simulink model "diagb"  (R2015a)
settings: Solver=ode45  StartTime=0.0  StopTime=10.0  RelTol=1e-3
settings Model: Creator=dayanm  LastModifiedBy=HP-14
settings OptimizationCC: ExpressionDepthLimit=2147483647
settings DebuggingCC: UnderspecifiedInitializationDetection=Classic  MergeDetectMultiDrivingBlocksExec=none  SolverPrmCheckMsg=warning  StateNameClashWarn=warning

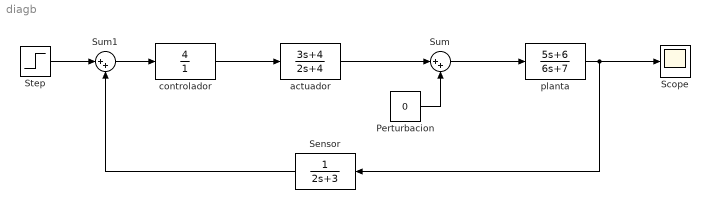
== system diagb ==
  Perturbacion : Constant  Value=0
  Scope : Scope
  Sensor : TransferFcn  Denominator=[2 3]
  Step : Step  SampleTime=0
  Sum : Sum  Inputs=|++
  Sum1 : Sum  Inputs=|++
  actuador : TransferFcn  Numerator=[3 4]  Denominator=[2 4]
  controlador : TransferFcn  Numerator=[4 ]  Denominator=[1]
  planta : TransferFcn  Numerator=[5 6]  Denominator=[6 7]
  wires:
  controlador/1 -> actuador/1
  Sum/1 -> planta/1
  actuador/1 -> Sum/1
  planta/1 -> Scope/1, Sensor/1
  Sensor/1 -> Sum1/2
  Sum1/1 -> controlador/1
  Step/1 -> Sum1/1
  Perturbacion/1 -> Sum/2
